simulink model "i2c_peripherals"  (R2016b)
settings: Solver=FixedStepDiscrete  StartTime=0.0  StopTime=10.0  FixedStep=.1  RelTol=1e-3
undefined symbols (not defined in the file): x1
libraries: mbed_lib x5, mbed_i2c_digital_io x5, mbed_i2c_analog_io x4, simulink x2, mbed_i2c_several x1, mbed_i2c_sensors x1
settings Model: Creator=Stuv  LastModifiedBy=oh
settings DataIOCC: LimitDataPoints=on  SaveFormat=Array
settings OptimizationCC: LifeSpan=1
settings DebuggingCC: SFUnexpectedBacktrackingDiag=warning  SFNoUnconditionalDefaultTransitionDiag=warning  SFExecutionAtInitializationDiag=none
settings HardwareCC: ProdBitPerPointer=32  ProdBitPerSizeT=32  ProdBitPerPtrDiffT=32  ProdLargestAtomicInteger=Long  ProdLargestAtomicFloat=Double  ProdIntDivRoundTo=Undefined  ProdWordSize=32  ProdHWDeviceType=ARM Compatible->ARM Cortex
settings ModelReferenceCC: PropagateSignalLabelsOutOfModel=off
settings RTWCC: SystemTargetFile=mbed.tlc  TemplateMakefile=mbed.tmf  Description=Mbed Target (Embedded Target)  TargetLang=C++
settings CodeAppCC: IgnoreCustomStorageClasses=off
settings STFCustomTargetCC: TargetLibSuffix=.a  GenerateSampleERTMain=on  CombineOutputUpdateFcns=on  ERTCustomFileBanners=on  SupportContinuousTime=off  SupportNonInlinedSFcns=off  RemoveResetFunc=on  MATLABClassNameForMDSCustomization=Simulink.SoftwareTarget.ERTCustomization  GRTInterface=off  SystemTargetFile=mbed.tlc
settings ERTTargetCC: GenerateSampleERTMain=on  ParMdlRefBuildCompliant=off  CompOptLevelCompliant=off  ConcurrentExecutionCompliant=off  ERTFirstTimeCompliant=off  ModelStepFunctionPrototypeControlCompliant=off  CPPClassGenCompliant=off  UseToolchainInfoCompliant=off  ERTCustomFileTemplate=mbed_file_process.tlc  ConvertIfToSwitch=off  SuppressUnreachableDefaultCases=off
settings ConfigComp: CovMetricSettings=dw  CovHtmlReporting=on  CovSaveCumulativeToWorkspaceVar=on  CovSaveSingleToWorkspaceVar=on  CovExternalEMLEnable=off

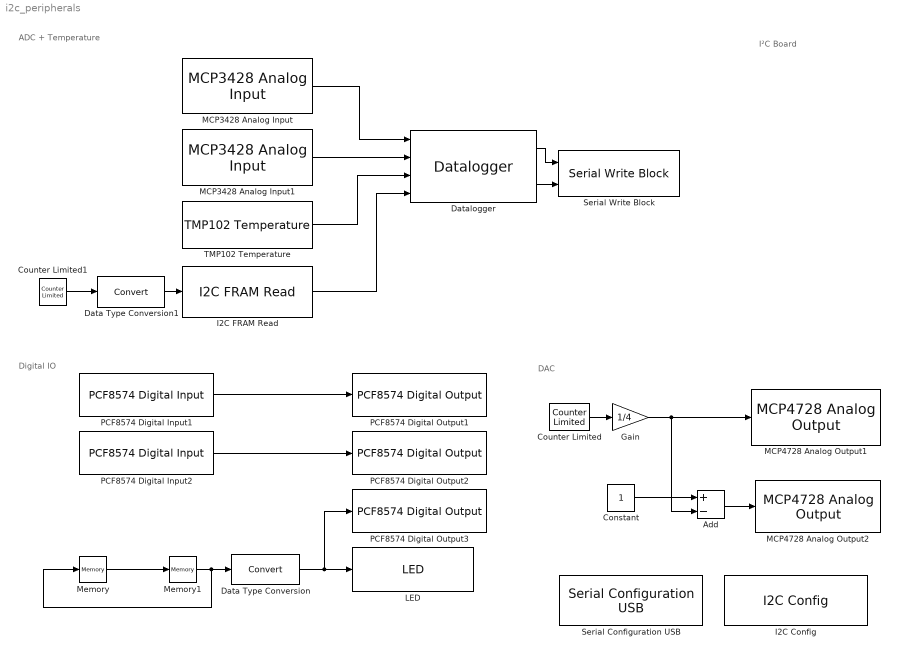
== system i2c_peripherals ==
  note: I²C Board
  note: Digital IO
  note: ADC + Temperature
  note: DAC
  Add : Sum  Inputs=+-
  Constant : Constant  OutDataTypeStr=single
  Counter Limited : simulink/Sources/Counter Limited  uplimit=4  tsamp=-1
  Counter Limited1 : simulink/Sources/Counter Limited  uplimit=11  tsamp=-1
  Data Type Conversion : DataTypeConversion
  Data Type Conversion1 : DataTypeConversion
  Datalogger : mbed_lib/Utilities/Datalogger  TypeInputPorts={ 'single' 1 'single' 1 'single' 1 'uint8' 1 }  TypeOfInputs={'1*single','1*single','1*single','1*uint8'}  BufferSize=40  errEn=off  SampleTime=-1
  Gain : Gain  Gain=1/4  OutDataTypeStr=single
  I2C Config : mbed_lib/Serial/I2C/I2C Config  Priority=0  I2CPort=1  Freq=100000  SDAPortName=B  SDAPinNumber=9  SCLPortName=B  SCLPinNumber=8
  I2C FRAM Read : mbed_i2c_several/I2C FRAM Read  I2cPort=1  EnableError=off
  LED : mbed_lib/GPIO/LED  nLED=1  SampleTime=-1
  MCP3428 Analog Input : mbed_i2c_analog_io/MCP3428 Analog Input  I2cPort=1  SubAddress=0xD0  EnableError=off  Channel=1  Mode=voltage  Resolution=12 bit  Gain=x1  SampleTime=-1
  MCP3428 Analog Input1 : mbed_i2c_analog_io/MCP3428 Analog Input  I2cPort=1  SubAddress=0xD2  EnableError=off  Channel=1  Mode=voltage  Resolution=12 bit  Gain=x1  SampleTime=-1
  MCP4728 Analog Output1 : mbed_i2c_analog_io/MCP4728 Analog Output  I2cPort=1  SubAddress=0xC0  EnableError=off  Channel=A  Mode=relative  RefVoltage=External  Gain=x1  SampleTime=-1
  MCP4728 Analog Output2 : mbed_i2c_analog_io/MCP4728 Analog Output  I2cPort=1  SubAddress=0xC0  EnableError=off  Channel=B  Mode=relative  RefVoltage=External  Gain=x1  SampleTime=-1
  Memory : Memory  X0=1  InheritSampleTime=on
  Memory1 : Memory  InheritSampleTime=on
  PCF8574 Digital Input1 : mbed_i2c_digital_io/PCF8574 Digital Input  I2cPort=1  SubAddress=0x40  PinNumber=Pin 6  EnableError=off  SampleTime=-1
  PCF8574 Digital Input2 : mbed_i2c_digital_io/PCF8574 Digital Input  I2cPort=1  SubAddress=0x72  PinNumber=Pin 7  EnableError=off  SampleTime=-1
  PCF8574 Digital Output1 : mbed_i2c_digital_io/PCF8574 Digital Output  I2cPort=1  SubAddress=0x40  PinNumber=Pin 0  EnableError=off  SampleTime=-1
  PCF8574 Digital Output2 : mbed_i2c_digital_io/PCF8574 Digital Output  I2cPort=1  SubAddress=0x40  PinNumber=Pin 1  EnableError=off  SampleTime=-1
  PCF8574 Digital Output3 : mbed_i2c_digital_io/PCF8574 Digital Output  I2cPort=1  SubAddress=0x40  PinNumber=Pin 2  EnableError=off  SampleTime=-1
  Serial Configuration USB : mbed_lib/Serial/UART/Serial Configuration USB  BaudRate=9600
  Serial Write Block : mbed_lib/Serial/UART/Serial Write Block  SerialPort=USB  numData=on  SampleTime=-1
  TMP102 Temperature : mbed_i2c_sensors/TMP102 Temperature  I2cPort=1  SubAddress=0x90  SampleRate=4 Hz  EnableError=off  SampleTime=-1
  wires:
  Datalogger/1 -> Serial Write Block/1
  Datalogger/2 -> Serial Write Block/2
  MCP3428 Analog Input1/1 -> Datalogger/2
  Memory/1 -> Memory1/1
  Memory1/1 -> Data Type Conversion/1, Memory/1
  Data Type Conversion/1 -> LED/1, PCF8574 Digital Output3/1
  TMP102 Temperature/1 -> Datalogger/3
  PCF8574 Digital Input2/1 -> PCF8574 Digital Output2/1
  PCF8574 Digital Input1/1 -> PCF8574 Digital Output1/1
  Counter Limited/1 -> Gain/1
  Gain/1 -> MCP4728 Analog Output1/1, Add/2
  Add/1 -> MCP4728 Analog Output2/1
  Constant/1 -> Add/1
  MCP3428 Analog Input/1 -> Datalogger/1
  Counter Limited1/1 -> Data Type Conversion1/1
  Data Type Conversion1/1 -> I2C FRAM Read/1
  I2C FRAM Read/1 -> Datalogger/4
